simulink model "ADRC_VoltageControl_Tuning"  (R2024b)
settings: Solver=ode23t  StartTime=0.0  StopTime=0.35  RelTol=1e-3
undefined symbols (not defined in the file): desired_dcMax, psu_V, Rload_Res, ts100us, VoltCtrlr_IGain, VoltCtrlr_PGain
libraries: fl_lib x5, nesl_utility x5, slctrl_adaptive x1, slpidlib x1
Description:
  | SEPIC Converter Voltage Control
settings Model: Creator=The MathWorks, Inc.  LastModifiedBy=vlenzi
settings DataIOCC: ExternalInput=getinputstruct(op1)  InitialState=getstatestruct(op1)  SignalLoggingName=adrcSim2
settings SimscapeCC: SimscapeLogType=all  SimscapeLogName=SepicVoltageControlSimlog  SimscapeLogLimitData=off

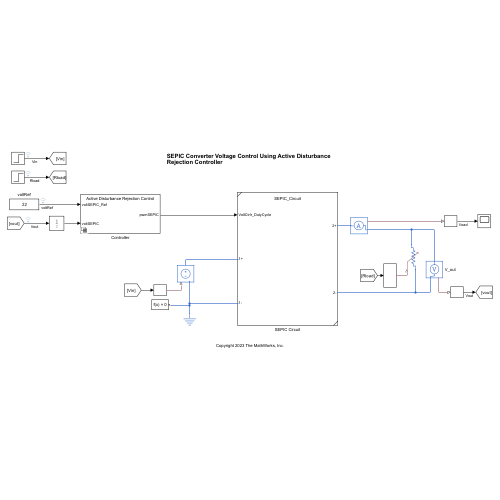
[thumbnail: Simulink's stored preview of the top-level diagram]
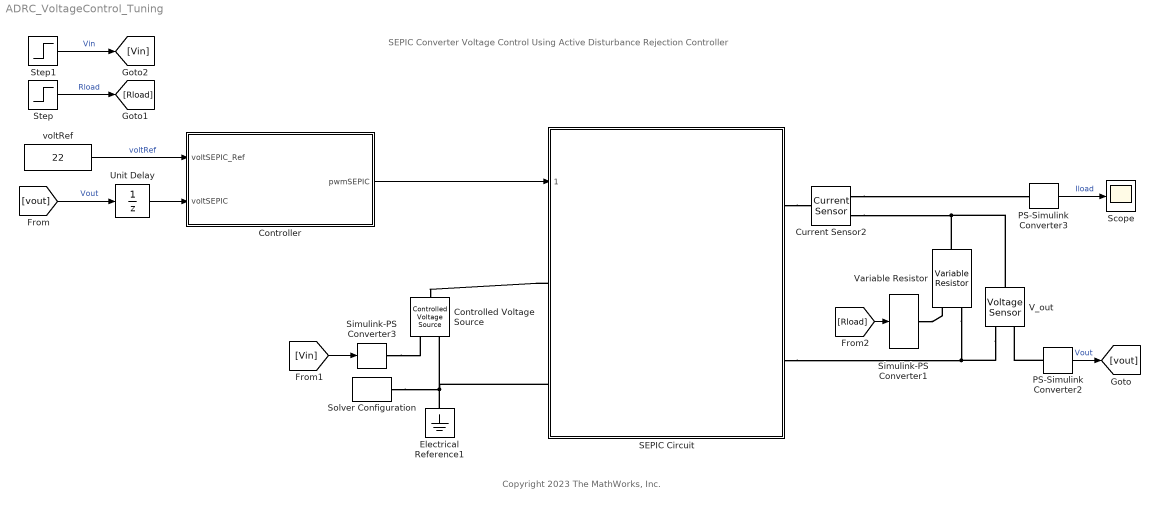
== system ADRC_VoltageControl_Tuning ==
  note: SEPIC Converter Voltage Control Using Active Disturbance Rejection Controller
  note: Copyright 2023 The MathWorks, Inc.
  Controlled Voltage Source : fl_lib/Electrical/Electrical Sources/Controlled Voltage Source
  Controller : Subsystem  Variant=on  VariantControlMode=label  VariantControl=control == 3  LabelModeActiveChoice=ADRC
  Current Sensor2 : fl_lib/Electrical/Electrical Sensors/Current Sensor
  Electrical Reference1 : fl_lib/Electrical/Electrical Elements/Electrical Reference
  PS-Simulink Converter2 : nesl_utility/PS-Simulink Converter  PhysicalDomain=network_engine_domain  SubClassName=ps_output  LeftPortType=input  RightPortType=output  PseudoPeriodic=off  Frequencies=[]  VectorFormat=1-D array  Unit=V  AffineConversion=off
  PS-Simulink Converter3 : nesl_utility/PS-Simulink Converter  PhysicalDomain=network_engine_domain  SubClassName=ps_output  LeftPortType=input  RightPortType=output  PseudoPeriodic=off  Frequencies=[]  VectorFormat=1-D array  Unit=mA  AffineConversion=off
  SEPIC Circuit : Subsystem  ReferencedSubsystem=SEPIC_Circuit
  Scope : Scope
  Simulink-PS Converter1 : nesl_utility/Simulink-PS Converter  PhysicalDomain=network_engine_domain  SubClassName=ps_input  LeftPortType=input  RightPortType=output  PseudoPeriodic=off  Frequencies=[]  NoiseDistribution=none  NoiseParameters=[]  Unit=1  AffineConversion=off  FilteringAndDerivatives=provide  SimscapeFilterOrder=1  InputFilterTimeConstant=1e-7  UdotUserProvided=0
  Simulink-PS Converter3 : nesl_utility/Simulink-PS Converter  PhysicalDomain=network_engine_domain  SubClassName=ps_input  LeftPortType=input  RightPortType=output  PseudoPeriodic=off  Frequencies=[]  NoiseDistribution=none  NoiseParameters=[]  Unit=1  AffineConversion=off  FilteringAndDerivatives=provide  SimscapeFilterOrder=1  InputFilterTimeConstant=1e-7  UdotUserProvided=0
  Solver Configuration : nesl_utility/Solver Configuration  PhysicalDomain=network_engine_domain  SubClassName=solver  LeftPortType=input  RightPortType=generic  Tones=[]  Harmonics=[]  SimulateNoise=off  Profile=off  UseLocalSampling=off  EnableSwitchedLinearOptims=on  FrequencyDomain=off  UseCCode=off  RelTol=0.001  AbsTol=1e-06  MinStep=1e-09  ToWorkspace=off  RevertToSquareIcSolve=off  NumHomotopyIterations=100  PhasorMode=off  PhasorModeNumHarmonics=1  ConsistencySolver=NEWTON_XTOL_AFTER_FTOL  IndexReductionMethod=DerivativeReplacement  DoDC=off  ResidualTolerance=1e-9  ConsistencyTolSource=GLOBAL  ConsistencyAbsTol=0.001  ConsistencyRelTol=0.001  ConsistencyTolFactor=0.001  UseLocalSolver=off  LocalSolverChoice=NE_BACKWARD_EULER_ADVANCER  ResolveIndetEquations=on  FunctionEvalNumThread=1  LocalSolverSampleTime=2e-7  DoFixedCost=off  MaxNonlinIter=2  MaxModeIter=2  ComputeImpulses=off  ImpulseIterations=2  LinearAlgebra=Sparse  LinearAlgebraNumThread=0  EquationFormulation=NE_TIME_EF  DelaysMemoryBudget=1024  AutomaticFiltering=on  FilteringTimeConstant=0.001  PartitionStorageMethod=AS_NEEDED  PartitionMemoryBudget=1024  PartitionMethod=ROBUST  MultibodyUseLocalSolver=off  MultibodyLocalSolverChoice=ODE1  MultibodyLocalSolverSampleTime=0.001
  Step : Step  Time=0.25  Before=Rload_Res  After=Rload_Res/2  SampleTime=0
  Step1 : Step  Time=0.15  Before=psu_V  After=psu_V+2  SampleTime=0
  Unit Delay : UnitDelay  SampleTime=-1  HasFrameUpgradeWarning=on
  V_out : fl_lib/Electrical/Electrical Sensors/Voltage Sensor
  Variable Resistor : fl_lib/Electrical/Electrical Elements/Variable Resistor  Rmin=0 Ohm  thermalEnable=false  thermal_mass=1 J/K  i_specify=off  i_priority=None  i=0 A  i_nominal_specify=off  i_nominal_value=1  i_nominal_unit=A  v_specify=off  v_priority=None  v=0 V  v_nominal_specify=off  v_nominal_value=1  v_nominal_unit=V  T_specify=off  T_priority=None  T=300 K  T_nominal_specify=off  T_nominal_value=1  T_nominal_unit=K
  voltRef : Constant  Value=22  SampleTime=0.001
  wires:
  voltRef/1 -> Controller/1(voltSEPIC_Ref)  "voltRef"
  Unit Delay/1 -> Controller/2(voltSEPIC)
  [vout] -> Unit Delay/1  "Vout"
  Step/1 -> [Rload]  "Rload"
  Step1/1 -> [Vin]  "Vin"
  PS-Simulink Converter3/1 -> Scope/1  "Iload"
  [Vin] -> Simulink-PS Converter3/1
  PS-Simulink Converter2/1 -> [vout]  "Vout"
  [Rload] -> Simulink-PS Converter1/1
  Controller/1(pwmSEPIC) -> SEPIC Circuit/1
  connections:
  Simulink-PS Converter1/RConn1 -- Variable Resistor/LConn1
  Current Sensor2/RConn1 -- PS-Simulink Converter3/LConn1
  SEPIC Circuit/LConn1 -- Controlled Voltage Source/LConn1
  PS-Simulink Converter2/LConn1 -- V_out/RConn1
  Simulink-PS Converter3/RConn1 -- Controlled Voltage Source/RConn1
  V_out/LConn1 -- Current Sensor2/RConn2 -- Variable Resistor/RConn1
  SEPIC Circuit/RConn1 -- Current Sensor2/LConn1
  Variable Resistor/LConn2 -- V_out/RConn2 -- SEPIC Circuit/RConn2
  Electrical Reference1/LConn1 -- Controlled Voltage Source/RConn2 -- SEPIC Circuit/LConn2 -- Solver Configuration/RConn1

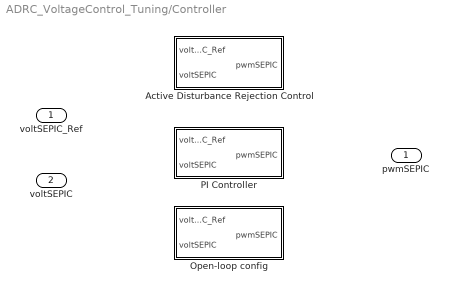
== system ADRC_VoltageControl_Tuning/Controller ==
  voltSEPIC_Ref : Inport
  voltSEPIC : Inport  Port=2
  Active Disturbance Rejection Control : Subsystem  VariantControl=ADRC
  Open-loop config : Subsystem  VariantControl=OpenLoop
  PI Controller : Subsystem  VariantControl=PI
  pwmSEPIC : Outport

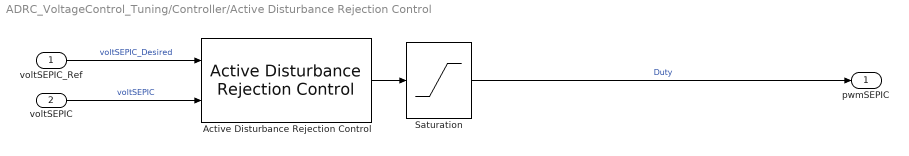
== system ADRC_VoltageControl_Tuning/Controller/Active Disturbance Rejection Control ==
  voltSEPIC_Ref : Inport
  voltSEPIC : Inport  Port=2
  Active Disturbance Rejection Control : slctrl_adaptive/Active Disturbance Rejection Control  time_domain=discrete-time  Ts=ts100us  model_type=second-order  b0=1.1903e7  wc=290  wo=290*7  x0=0  ulim_checkbox=on  umax=0.99  umin=0.01  xhat_checkbox=off
      settings: LibrarySourceBlock=slctrlblks/Adaptive Control/Active Disturbance Rejection Control
  Saturation : Saturate  UpperLimit=desired_dcMax  LowerLimit=0
      settings: AttributesFormatString=|
      | %<UpperLimit>
      | %<LowerLimit>
  pwmSEPIC : Outport
  wires:
  Active Disturbance Rejection Control/1 -> Saturation/1
  voltSEPIC/1 -> Active Disturbance Rejection Control/2  "voltSEPIC"
  voltSEPIC_Ref/1 -> Active Disturbance Rejection Control/1  "voltSEPIC_Desired"
  Saturation/1 -> pwmSEPIC/1  "Duty"

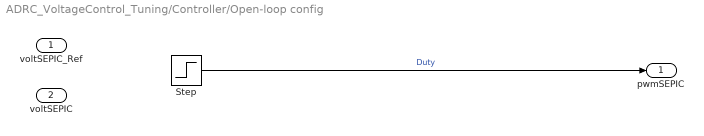
== system ADRC_VoltageControl_Tuning/Controller/Open-loop config ==
  voltSEPIC_Ref : Inport
  voltSEPIC : Inport  Port=2
  Step : Step  Time=0  After=0.62  SampleTime=0
  pwmSEPIC : Outport
  wires:
  Step/1 -> pwmSEPIC/1  "Duty"

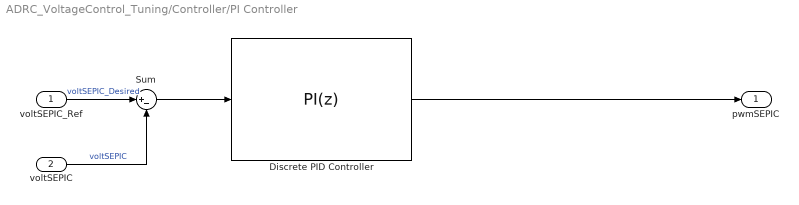
== system ADRC_VoltageControl_Tuning/Controller/PI Controller ==
  voltSEPIC_Ref : Inport
  voltSEPIC : Inport  Port=2
  Discrete PID Controller : slpidlib/PID Controller  Controller=PI  Form=Parallel  TimeDomain=Discrete-time  UseExternalTs=off  SampleTime=ts100us  IntegratorMethod=Forward Euler  FilterMethod=Forward Euler  ControllerParametersSource=internal  P=double(VoltCtrlr_PGain)  I=double(VoltCtrlr_IGain)  UseKiTs=off  D=0  UseExternalDerivativeSource=off  N=100  UseFilter=on  TunerSelectOption=Transfer Function Based (PID Tuner App)  InitialConditionSource=internal  InitialConditionForIntegrator=0  InitialConditionForFilter=0  DifferentiatorICPrevScaledInput=0  ExternalReset=none  TrackingMode=off  Kt=1  LimitOutput=on  SatLimitsSource=internal  UpperSaturationLimit=desired_dcMax  LowerSaturationLimit=0  LinearizeAsGain=off  AntiWindupMode=clamping  Kb=1  LimitIntegrator=off  UpperIntegratorSaturationLimit=inf  LowerIntegratorSaturationLimit=-inf  POutMin=[]  POutMax=[]  IOutMin=[]  IOutMax=[]  DOutMin=[]  DOutMax=[]  NOutMin=[]  NOutMax=[]  SumOutMin=[]  SumOutMax=[]  SaturationOutMin=[]  SaturationOutMax=[]  PParamMin=[]  PParamMax=[]  IParamMin=[]  IParamMax=[]  DParamMin=[]  DParamMax=[]  NParamMin=[]  NParamMax=[]  KbParamMin=[]  KbParamMax=[]  KtParamMin=[]  KtParamMax=[]  KbOutMin=[]  KbOutMax=[]  KtOutMin=[]  KtOutMax=[]  IntegratorOutMin=[]  IntegratorOutMax=[]  FilterOutMin=[]  FilterOutMax=[]  SumI1OutMin=[]  SumI1OutMax=[]  SumI2OutMin=[]  SumI2OutMax=[]  SumI3OutMin=[]  SumI3OutMax=[]  SumI4OutMin=[]  SumI4OutMax=[]  SumDOutMin=[]  SumDOutMax=[]  DifferentiatorOutMin=[]  DifferentiatorOutMax=[]  FilterDiffOutCoefMin=[]  FilterDiffOutCoefMax=[]  ReciprocalOutMin=[]  ReciprocalOutMax=[]  SumDenOutMin=[]  SumDenOutMax=[]  SumNumOutMin=[]  SumNumOutMax=[]  DivideOutMin=[]  DivideOutMax=[]  UdiffTsProdOutMin=[]  UdiffTsProdOutMax=[]  NTsProdOutMin=[]  NTsProdOutMax=[]  UintegralTsProdOutMin=[]  UintegralTsProdOutMax=[]  UngainTsProdOutMin=[]  UngainTsProdOutMax=[]  ClampingZeroOutDataTypeStr=Inherit: Inherit via back propagation  ClampingZeroOutMin=[]  ClampingZeroOutMax=[]  FilterDenConstantOutDataTypeStr=Inherit: Inherit via back propagation  FilterDenConstantOutMin=[]  FilterDenConstantOutMax=[]  PCopyOutDataTypeStr=Inherit: Inherit via back propagation  PCopyOutMin=[]  PCopyOutMax=[]  NCopyOutDataTypeStr=Inherit: Inherit via back propagation  NCopyOutMin=[]  NCopyOutMax=[]  IntegratorContinuousStateAttributes=''  IntegratorStateMustResolveToSignalObject=off  IntegratorRTWStateStorageClass=Auto  FilterContinuousStateAttributes=''  FilterStateMustResolveToSignalObject=off  FilterRTWStateStorageClass=Auto  ParallelPVariant=InternalParameters  IdealPVariant=Disabled  IVariant=InternalParameters  DVariant=Disabled  IntegratorVariant=Discrete  SatVariant=Enabled  AWVariant=DiscClampingParallel  PCopyVariant=Disabled  TRVariant=Disabled  FdbkBlocksVariant=Forward  IdealPFdbkVariant=Disabled  SatFdbkVariant=Disabled  DerivativeFilterVariant=Disabled  NVariant=Disabled  NCopyVariant=Disabled_SignalSpec  FilterICVariant=Disabled  IntegratorICVariant=InternalICs  ExternalResetVariant=Disabled  TRSumVariant=Passthrough  SumFdbkVariant=Disabled  SumVariant=Sum_PI  TsampFilterVariant=InternalTs  TsampNgainVariant=Passthrough  TsampIntegralVariant=Disabled_SignalSpec  ExternalSaturationOutDataTypeStr=Inherit: Same as second input  DerivativeSourceVariant=Disabled  PreIntVariant=InternalPreInt
  Sum : Sum  Inputs=|+-
  pwmSEPIC : Outport
  wires:
  Sum/1 -> Discrete PID Controller/1
  voltSEPIC/1 -> Sum/2  "voltSEPIC"
  Discrete PID Controller/1 -> pwmSEPIC/1
  voltSEPIC_Ref/1 -> Sum/1  "voltSEPIC_Desired"
